simulink model "Pacemaker_Assignment1_group33"  (R2020a)
settings: Solver=FixedStepAuto  StartTime=0.0  StopTime=10.0  FixedStep=1e-3  RelTol=1e-3  EnableMultiTasking=on
undefined symbols (not defined in the file): D0, D1, D10, D11, D12, D13, D2, D3, D4, D5, D6, D7, D8, D9, PTA0, PTA1, PTA2, PTB23, PTB9, PTC16, PTC17, PTC2, PTC3, PTC4, PTD0, PTD1, PTD2, PTD3
libraries: frdmk64flib x16
settings Model: ExtModeTrigDuration=5  Creator=sxj  LastModifiedBy=sxj
settings OptimizationCC: EnhancedBackFolding=on  PassReuseOutputArgsAs=Individual arguments  ZeroExternalMemoryAtStartup=off  ZeroInternalMemoryAtStartup=off  MaxStackSize=64  OptimizeBlockOrder=speed  DifferentSizesBufferReuse=on  OptimizationCustomize=off  EfficientTunableParamExpr=on
settings DebuggingCC: ParameterTunabilityLossMsg=error
settings HardwareCC: ProdBitPerPointer=32  ProdBitPerSizeT=32  ProdBitPerPtrDiffT=32  ProdLargestAtomicInteger=Long  ProdLargestAtomicFloat=Double  ProdWordSize=32  ProdHWDeviceType=ARM Compatible->ARM Cortex
settings SFSimCC: MATLABDynamicMemAlloc=off
settings RTWCC: SystemTargetFile=ert.tlc  HardwareBoard=NXP FRDM-K64F  TemplateMakefile=ert_default_tmf  Toolchain=GNU Tools for ARM Embedded Processors
settings CodeAppCC: ForceParamTrailComments=on  IgnoreCustomStorageClasses=off  OperatorAnnotations=on  SimulinkDataObjDesc=on  SFDataObjDesc=on  InsertBlockDesc=on

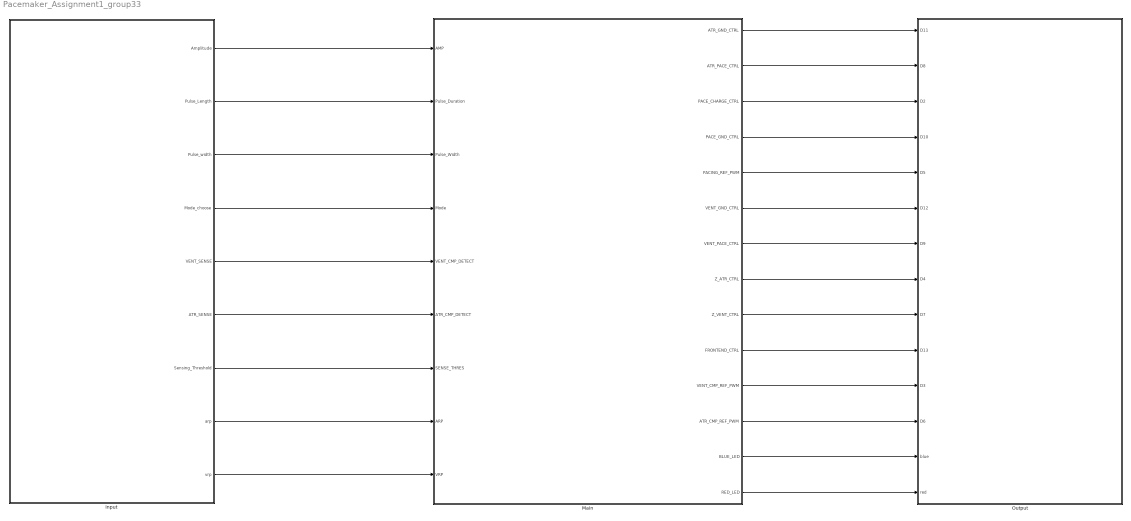
== system Pacemaker_Assignment1_group33 ==
  Input : Subsystem
  Main : Stateflow chart  TreatAsAtomicUnit=on
  Output : Subsystem
  wires:
  Input/1(Amplitude) -> Main/1(AMP)
  Input/2(Pulse_Length) -> Main/2(Pulse_Duration)
  Input/3(Pulse_width) -> Main/3(Pulse_Width)
  Input/4(Mode_choose) -> Main/4(Mode)
  Input/5(VENT_SENSE) -> Main/5(VENT_CMP_DETECT)
  Input/6(ATR_SENSE) -> Main/6(ATR_CMP_DETECT)
  Input/7(Sensing_Threshold) -> Main/7(SENSE_THRES)
  Main/1(ATR_GND_CTRL) -> Output/1(D11)
  Main/2(ATR_PACE_CTRL) -> Output/2(D8)
  Main/3(PACE_CHARGE_CTRL) -> Output/3(D2)
  Main/4(PACE_GND_CTRL) -> Output/4(D10)
  Main/5(PACING_REF_PWM) -> Output/5(D5)
  Main/6(VENT_GND_CTRL) -> Output/6(D12)
  Main/7(VENT_PACE_CTRL) -> Output/7(D9)
  Main/8(Z_ATR_CTRL) -> Output/8(D4)
  Main/9(Z_VENT_CTRL) -> Output/9(D7)
  Main/10(FRONTEND_CTRL) -> Output/10(D13)
  Main/11(VENT_CMP_REF_PWM) -> Output/11(D3)
  Main/12(ATR_CMP_REF_PWM) -> Output/12(D6)
  Main/13(BLUE_LED) -> Output/13(blue)
  Main/14(RED_LED) -> Output/14(red)
  Input/8(arp) -> Main/8(ARP)
  Input/9(vrp) -> Main/9(VRP)

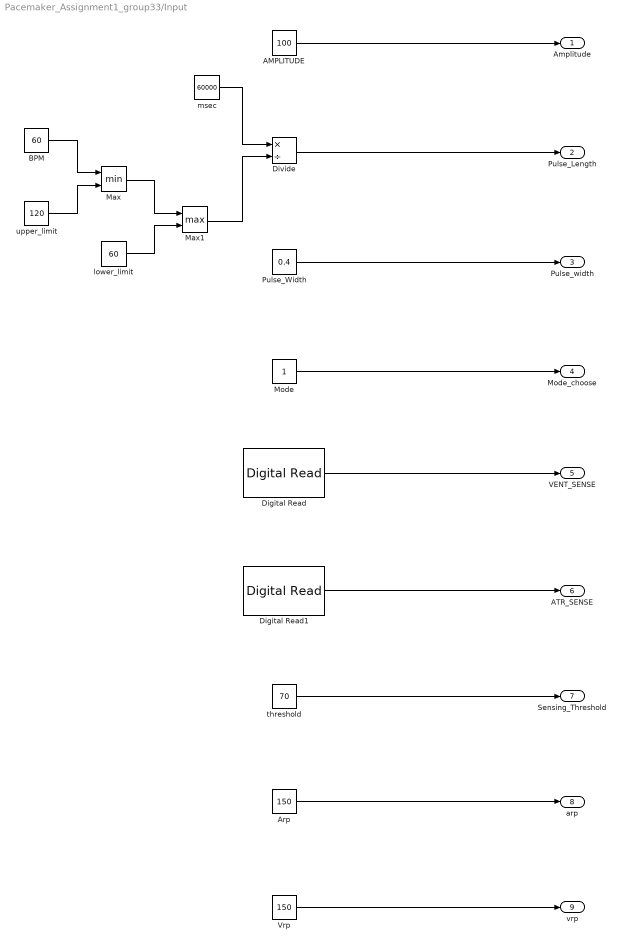
== system Pacemaker_Assignment1_group33/Input ==
  AMPLITUDE : Constant  Value=100
  Arp : Constant  Value=150
  BPM : Constant  Value=60
  Digital Read : frdmk64flib/Digital Read  Whichpin=PTC17 (D1)  SampleTime=-1
  Digital Read1 : frdmk64flib/Digital Read  Whichpin=PTC16 (D0)  SampleTime=-1
  Divide : Product  Inputs=*/
  Max : MinMax  Inputs=2
  Max1 : MinMax  Function=max  Inputs=2
  Mode : Constant
  Pulse_Width : Constant  Value=0.4
  Vrp : Constant  Value=150
  lower_limit : Constant  Value=60
  msec : Constant  Value=60000
  threshold : Constant  Value=70
  upper_limit : Constant  Value=120
  Amplitude : Outport
  Pulse_Length : Outport  Port=2
  Pulse_width : Outport  Port=3
  Mode_choose : Outport  Port=4
  VENT_SENSE : Outport  Port=5
  ATR_SENSE : Outport  Port=6
  Sensing_Threshold : Outport  Port=7
  arp : Outport  Port=8
  vrp : Outport  Port=9
  wires:
  Max1/1 -> Divide/2
  msec/1 -> Divide/1
  AMPLITUDE/1 -> Amplitude/1
  Divide/1 -> Pulse_Length/1
  Pulse_Width/1 -> Pulse_width/1
  Mode/1 -> Mode_choose/1
  Digital Read/1 -> VENT_SENSE/1
  Digital Read1/1 -> ATR_SENSE/1
  threshold/1 -> Sensing_Threshold/1
  Arp/1 -> arp/1
  Vrp/1 -> vrp/1
  lower_limit/1 -> Max1/2
  Max/1 -> Max1/1
  upper_limit/1 -> Max/2
  BPM/1 -> Max/1

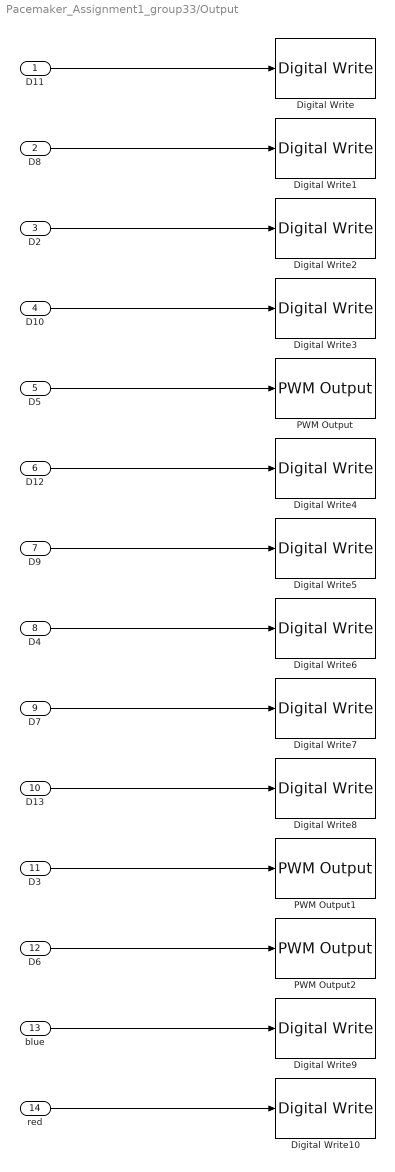
== system Pacemaker_Assignment1_group33/Output ==
  D11 : Inport
  D8 : Inport  Port=2
  D2 : Inport  Port=3
  D10 : Inport  Port=4
  D5 : Inport  Port=5
  D12 : Inport  Port=6
  D9 : Inport  Port=7
  D4 : Inport  Port=8
  D7 : Inport  Port=9
  D13 : Inport  Port=10
  D3 : Inport  Port=11
  D6 : Inport  Port=12
  blue : Inport  Port=13
  red : Inport  Port=14
  Digital Write : frdmk64flib/Digital Write  Whichpin=PTD2 (D11)
  Digital Write1 : frdmk64flib/Digital Write  Whichpin=PTA0 (D8)
  Digital Write10 : frdmk64flib/Digital Write  Whichpin=RED_LED
  Digital Write2 : frdmk64flib/Digital Write  Whichpin=PTB9 (D2)
  Digital Write3 : frdmk64flib/Digital Write  Whichpin=PTD0 (D10)
  Digital Write4 : frdmk64flib/Digital Write  Whichpin=PTD3 (D12)
  Digital Write5 : frdmk64flib/Digital Write  Whichpin=PTC4 (D9)
  Digital Write6 : frdmk64flib/Digital Write  Whichpin=PTB23 (D4)
  Digital Write7 : frdmk64flib/Digital Write  Whichpin=PTC3 (D7)
  Digital Write8 : frdmk64flib/Digital Write  Whichpin=PTD1 (D13)
  Digital Write9 : frdmk64flib/Digital Write  Whichpin=BLUE_LED
  PWM Output : frdmk64flib/PWM Output  Whichpin=PTA2 (D5)  InitialFrequency=2000  InitialDutyCycle=0
  PWM Output1 : frdmk64flib/PWM Output  Whichpin=PTA1 (D3)  InitialFrequency=2000  InitialDutyCycle=0
  PWM Output2 : frdmk64flib/PWM Output  Whichpin=PTC2 (D6)  InitialFrequency=2000  InitialDutyCycle=0
  wires:
  D11/1 -> Digital Write/1
  D8/1 -> Digital Write1/1
  D2/1 -> Digital Write2/1
  D10/1 -> Digital Write3/1
  D5/1 -> PWM Output/1
  D12/1 -> Digital Write4/1
  D9/1 -> Digital Write5/1
  D4/1 -> Digital Write6/1
  D7/1 -> Digital Write7/1
  D13/1 -> Digital Write8/1
  D3/1 -> PWM Output1/1
  D6/1 -> PWM Output2/1
  blue/1 -> Digital Write9/1
  red/1 -> Digital Write10/1

== stateflow chart Pacemaker_Assignment1_group33/Main ==
  state AOO
    state AOO_CHARGE
      entry:
      PACING_REF_PWM = AMP;
      PACE_CHARGE_CTRL = 1;
      ATR_PACE_CTRL = 0;
      ATR_GND_CTRL = 1;
      PACE_GND_CTRL = 1;
      Z_ATR_CTRL = 0;
      VENT_PACE_CTRL = 0;
      VENT_GND_CTRL = 0;
      Z_VENT_CTRL = 0;
      BLUE_LED = 0;
      RED_LED = 1;
    state AOO_PACE
      entry:
      PACING_REF_PWM = AMP;
      PACE_CHARGE_CTRL = 0;
      ATR_PACE_CTRL = 1;
      ATR_GND_CTRL = 0;
      PACE_GND_CTRL = 1;
      Z_ATR_CTRL = 0;
      VENT_PACE_CTRL = 0;
      VENT_GND_CTRL = 0;
      Z_VENT_CTRL = 0;
      BLUE_LED = 1;
      RED_LED = 0;
    (default) -> AOO_CHARGE
    AOO_CHARGE -> AOO_PACE : after(Pulse_Duration-Pulse_Width,msec)
    AOO_PACE -> AOO_CHARGE : after(Pulse_Width,msec)
  state VVI
    state VVI_CHARGE
      entry:
      PACING_REF_PWM = AMP;
      PACE_CHARGE_CTRL = 1;
      VENT_PACE_CTRL = 0;
      VENT_GND_CTRL = 1;
      PACE_GND_CTRL = 1;
      Z_VENT_CTRL = 0;
      FRONTEND_CTRL = 1;
      VENT_CMP_REF_PWM = SENSE_THRES;
      ATR_PACE_CTRL = 0;
      ATR_GND_CTRL = 0;
      Z_ATR_CTRL = 0;
    state VVI_PACE
      entry:
      PACING_REF_PWM = AMP;
      PACE_CHARGE_CTRL = 0;
      VENT_PACE_CTRL = 1;
      VENT_GND_CTRL = 0;
      PACE_GND_CTRL = 1;
      Z_VENT_CTRL = 0;
      FRONTEND_CTRL = 1;
      VENT_CMP_REF_PWM = SENSE_THRES;
      ATR_PACE_CTRL = 0;
      ATR_GND_CTRL = 0;
      Z_ATR_CTRL = 0;
    (junction 55) -> VVI_CHARGE [order 2] : [VENT_CMP_DETECT == 1]
    (default) -> VVI_CHARGE
    VVI_CHARGE -> (junction 55) : after(VRP,msec)
    (junction 55) -> VVI_PACE [order 1] : after(Pulse_Duration-VRP-Pulse_Width,msec)[VENT_CMP_DETECT == 0]
    VVI_PACE -> VVI_CHARGE : after(Pulse_Width,msec)
  state AAI
    state AAI_PACE
      entry:
      PACING_REF_PWM = AMP;
      PACE_CHARGE_CTRL = 0;
      ATR_PACE_CTRL = 1;
      ATR_GND_CTRL = 0;
      PACE_GND_CTRL = 1;
      Z_ATR_CTRL = 0;
      FRONTEND_CTRL = 1;
      ATR_CMP_REF_PWM = SENSE_THRES;
      VENT_PACE_CTRL = 0;
      VENT_GND_CTRL = 0;
      Z_VENT_CTRL = 0;
    state AAI_CHARGE
      entry:
      PACING_REF_PWM = AMP;
      PACE_CHARGE_CTRL = 1;
      ATR_PACE_CTRL = 0;
      ATR_GND_CTRL = 1;
      PACE_GND_CTRL = 1;
      Z_ATR_CTRL = 0;
      FRONTEND_CTRL = 1;
      ATR_CMP_REF_PWM = SENSE_THRES;
      VENT_PACE_CTRL = 0;
      VENT_GND_CTRL = 0;
      Z_VENT_CTRL = 0;
    (junction 49) -> AAI_CHARGE [order 2] : [ATR_CMP_DETECT == 1]
    (default) -> AAI_CHARGE
    AAI_CHARGE -> (junction 49) : after(ARP,msec)
    (junction 49) -> AAI_PACE [order 1] : after(Pulse_Duration-ARP-Pulse_Width,msec)[ATR_CMP_DETECT == 0]
    AAI_PACE -> AAI_CHARGE : after(Pulse_Width,msec)
  state IDLE_STATE
  state VOO
    state VOO_CHARGE
      entry:
      PACING_REF_PWM = AMP;
      PACE_CHARGE_CTRL = 1;
      VENT_PACE_CTRL = 0;
      VENT_GND_CTRL = 1;
      PACE_GND_CTRL = 1;
      Z_VENT_CTRL = 0;
      ATR_PACE_CTRL = 0;
      ATR_GND_CTRL = 0;
      Z_ATR_CTRL = 0;
      BLUE_LED = 0;
      RED_LED = 1;
    state VOO_PACE
      entry:
      PACING_REF_PWM = AMP;
      PACE_CHARGE_CTRL = 0;
      VENT_PACE_CTRL = 1;
      VENT_GND_CTRL = 0;
      PACE_GND_CTRL = 1;
      Z_VENT_CTRL = 0;
      ATR_PACE_CTRL = 0;
      ATR_GND_CTRL = 0;
      Z_ATR_CTRL = 0;
      BLUE_LED = 1;
      RED_LED = 0;
    (default) -> VOO_CHARGE
    VOO_CHARGE -> VOO_PACE : after(Pulse_Duration-Pulse_Width,msec)
    VOO_PACE -> VOO_CHARGE : after(Pulse_Width,msec)
  IDLE_STATE -> AOO [order 1] : [Mode == 0]
  AOO -> IDLE_STATE : [Mode ~= 0]
  (default) -> IDLE_STATE
  IDLE_STATE -> VVI [order 4] : [Mode == 3]
  IDLE_STATE -> AAI [order 3] : [Mode == 2]
  AAI -> IDLE_STATE : [Mode ~= 2]
  VVI -> IDLE_STATE : [Mode ~= 3]
  IDLE_STATE -> VOO [order 2] : [Mode == 1]
  VOO -> IDLE_STATE : [Mode ~= 1]
  data: AMP input; ATR_GND_CTRL output; ATR_PACE_CTRL output; PACE_CHARGE_CTRL output; PACE_GND_CTRL output; PACING_REF_PWM output; VENT_GND_CTRL output; VENT_PACE_CTRL output; Z_ATR_CTRL output; Z_VENT_CTRL output; Pulse_Duration input; Pulse_Width input; Mode input; FRONTEND_CTRL output; VENT_CMP_DETECT input; ATR_CMP_DETECT input; SENSE_THRES input; VENT_CMP_REF_PWM output; ATR_CMP_REF_PWM output; BLUE_LED output; RED_LED output; ARP input; VRP input
